simulink model "Task_7"  (R2017a)
settings: Solver=VariableStepAuto  StartTime=0.0  StopTime=10.0  MaxStep=0.001  RelTol=1e-3
libraries: simulink x2
settings Model: Creator=HP  LastModifiedBy=User

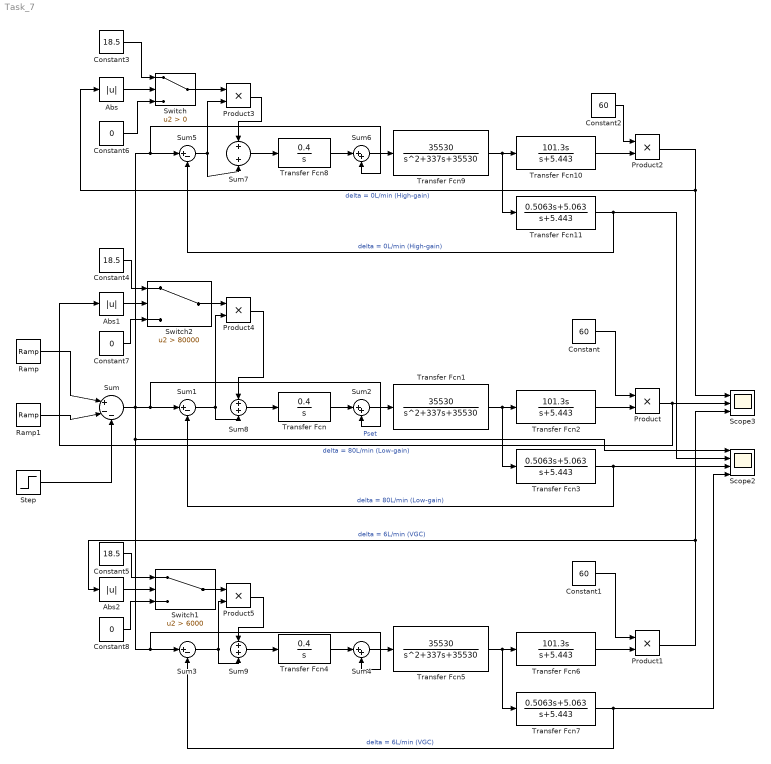
== system Task_7 ==
  Abs : Abs  SaturateOnIntegerOverflow=off
  Abs1 : Abs  SaturateOnIntegerOverflow=off
  Abs2 : Abs  SaturateOnIntegerOverflow=off
  Constant : Constant  Value=60
  Constant1 : Constant  Value=60
  Constant2 : Constant  Value=60
  Constant3 : Constant  Value=18.5
  Constant4 : Constant  Value=18.5
  Constant5 : Constant  Value=18.5
  Constant6 : Constant  Value=0
  Constant7 : Constant  Value=0
  Constant8 : Constant  Value=0
  Product{,1..5} (6 alike) : Product
  Ramp : simulink/Sources/Ramp  slope=64.9351  start=0  X0=0
  Ramp1 : simulink/Sources/Ramp  slope=64.9531  start=0.231  X0=0
  Scope2 : Scope  NumInputPorts=4
  Scope3 : Scope  NumInputPorts=3
  Step : Step  Time=4  After=15  SampleTime=0
  Sum : Sum  Inputs=|+--
  Sum1 : Sum  Inputs=|+-
  Sum2 : Sum  Inputs=|++
  Sum3 : Sum  Inputs=|+-
  Sum4 : Sum  Inputs=|++
  Sum5 : Sum  Inputs=|+-
  Sum6 : Sum  Inputs=|++
  Sum7 : Sum
  Sum8 : Sum
  Sum9 : Sum
  Switch : Switch  Criteria=u2 > Threshold  SaturateOnIntegerOverflow=off  InputSameDT=off
  Switch1 : Switch  Criteria=u2 > Threshold  Threshold=6000  SaturateOnIntegerOverflow=off  InputSameDT=off
  Switch2 : Switch  Criteria=u2 > Threshold  Threshold=80000  SaturateOnIntegerOverflow=off  InputSameDT=off
  Transfer Fcn : TransferFcn  Numerator=[0.4]  Denominator=[1 0]
  Transfer Fcn1 : TransferFcn  Numerator=[35530]  Denominator=[1 337 35530]
  Transfer Fcn10 : TransferFcn  Numerator=[101.3 0]  Denominator=[1 5.443]
  Transfer Fcn11 : TransferFcn  Numerator=[0.5063 5.063]  Denominator=[1 5.443]
  Transfer Fcn2 : TransferFcn  Numerator=[101.3 0]  Denominator=[1 5.443]
  Transfer Fcn3 : TransferFcn  Numerator=[0.5063 5.063]  Denominator=[1 5.443]
  Transfer Fcn4 : TransferFcn  Numerator=[0.4]  Denominator=[1 0]
  Transfer Fcn5 : TransferFcn  Numerator=[35530]  Denominator=[1 337 35530]
  Transfer Fcn6 : TransferFcn  Numerator=[101.3 0]  Denominator=[1 5.443]
  Transfer Fcn7 : TransferFcn  Numerator=[0.5063 5.063]  Denominator=[1 5.443]
  Transfer Fcn8 : TransferFcn  Numerator=[0.4]  Denominator=[1 0]
  Transfer Fcn9 : TransferFcn  Numerator=[35530]  Denominator=[1 337 35530]
  wires:
  Product2/1 -> Abs/1, Scope3/1  "delta = 0L/min (High-gain)"
  Ramp1/1 -> Sum/2
  Step/1 -> Sum/3
  Sum/1 -> Scope2/1, Sum4/2, Sum3/1, Sum6/2, Sum5/1, Sum2/2, Sum1/1  "Pset"
  Transfer Fcn1/1 -> Transfer Fcn3/1, Transfer Fcn2/1
  Sum2/1 -> Transfer Fcn1/1
  Product1/1 -> Abs2/1, Scope3/3  "delta = 6L/min (VGC)"
  Constant/1 -> Product/1
  Transfer Fcn3/1 -> Scope2/3, Sum1/2  "delta = 80L/min (Low-gain)"
  Transfer Fcn5/1 -> Transfer Fcn7/1, Transfer Fcn6/1
  Sum4/1 -> Transfer Fcn5/1
  Transfer Fcn4/1 -> Sum4/1
  Transfer Fcn2/1 -> Product/2
  Constant1/1 -> Product1/1
  Transfer Fcn/1 -> Sum2/1
  Transfer Fcn11/1 -> Scope2/2, Sum5/2  "delta = 0L/min (High-gain)"
  Transfer Fcn7/1 -> Scope2/4, Sum3/2  "delta = 6L/min (VGC)"
  Product/1 -> Abs1/1, Scope3/2  "delta = 80L/min (Low-gain)"
  Transfer Fcn6/1 -> Product1/2
  Transfer Fcn9/1 -> Transfer Fcn11/1, Transfer Fcn10/1
  Sum6/1 -> Transfer Fcn9/1
  Transfer Fcn10/1 -> Product2/2
  Transfer Fcn8/1 -> Sum6/1
  Constant2/1 -> Product2/1
  Ramp/1 -> Sum/1
  Sum8/1 -> Transfer Fcn/1
  Sum9/1 -> Transfer Fcn4/1
  Sum3/1 -> Product5/2, Sum9/2
  Sum1/1 -> Product4/2, Sum8/2
  Sum7/1 -> Transfer Fcn8/1
  Sum5/1 -> Sum7/2, Product3/2
  Product3/1 -> Sum7/1
  Switch/1 -> Product3/1
  Abs/1 -> Switch/2
  Product4/1 -> Sum8/1
  Switch2/1 -> Product4/1
  Abs1/1 -> Switch2/2
  Product5/1 -> Sum9/1
  Switch1/1 -> Product5/1
  Abs2/1 -> Switch1/2
  Constant3/1 -> Switch/1
  Constant5/1 -> Switch1/1
  Constant4/1 -> Switch2/1
  Constant6/1 -> Switch/3
  Constant7/1 -> Switch2/3
  Constant8/1 -> Switch1/3
